simulink model "suspension_3dof"  (R2022b)
settings: Solver=ode45  StartTime=0.0  StopTime=100  MaxStep=0.001  RelTol=1e-3  AbsTol=1e-6
PreLoadFcn:
  | sldemo_suspn_3dof_data
values from neighbouring files (symbols this model uses):
  Cr = 2000    [sldemo_suspn_3dof_data.m]
  g = 9.81    [sldemo_suspn_3dof_data.m]
  Ixx = 1500    [sldemo_suspn_3dof_data.m]
  Iyy = 2100    [sldemo_suspn_3dof_data.m]
  Kf = 28000    [sldemo_suspn_3dof_data.m]
  Kr = 21000    [sldemo_suspn_3dof_data.m]
  L = 1.2    [sldemo_suspn_3dof_data.m]
  Mb = 1200    [sldemo_suspn_3dof_data.m]
  W = 0.9    [sldemo_suspn_3dof_data.m]
libraries: SignalEditorBlockLib x1
CloseFcn:
  | clear Cf Cr Ixx Iyy Kf Kr L Mb W g x0;
Description:
  | Automotive Suspension
  | 
  | This demo describes a simplified car suspension model in three degrees of
  | freedom (DoF): pitch, yaw and vertical displacement. The demo provides a description of the model to
  | show how simulation can be used for investigating ride characteristics. The Signal Editor block was used to
  | capture different road profiles to test the suspension against.
settings Model: FPTRunName=Active  ModifiedByFormat=The MathWorks Inc.  TunableVars=Cf,Mb  TunableVarsStorageClass=Auto,Auto  TunableVarsTypeQualifier=,  Creator=The MathWorks, Inc.  LastModifiedBy=The MathWorks Inc.
settings SolverCC: AutoScaleAbsTol=off  AlgebraicLoopSolver=TrustRegion
settings DataIOCC: InitialState=x0  SaveFormat=Array  SaveOutput=off  DSMLogging=off  SaveTime=off  StateSaveName=x  ReturnWorkspaceOutputsName=simout
settings OptimizationCC: BooleanDataType=off  DefaultParameterBehavior=Inlined  InlineInvariantSignals=on  ExpressionDepthLimit=2147483647  InitFltsAndDblsToZero=on  LifeSpan=inf  BufferReusableBoundary=off
settings DebuggingCC: SaveWithParameterizedLinksMsg=none  SignalResolutionControl=TryResolveAllWithWarning  MultiTaskDSMMsg=warning  SigSpecEnsureSampleTimeMsg=none  IntegerOverflowMsg=none  FcnCallInpInsideContextMsg=warning  UnconnectedInputMsg=warning  UnconnectedOutputMsg=warning  UnconnectedLineMsg=warning  BusObjectLabelMismatch=none  StateNameClashWarn=warning  PregeneratedLibrarySubsystemCodeDiagnostic=none  SFUnexpectedBacktrackingDiag=warning  SFNoUnconditionalDefaultTransitionDiag=warning  SFExecutionAtInitializationDiag=none  SFMachineParentedDataDiag=warning  IntegerSaturationMsg=none  ArithmeticOperatorsInVariantConditions=warning
settings HardwareCC: ProdBitPerPointer=32  ProdBitPerSizeT=32  ProdBitPerPtrDiffT=32  ProdLargestAtomicFloat=None  ProdIntDivRoundTo=Undefined  ProdEndianess=Unspecified  ProdWordSize=32  ProdHWDeviceType=32-bit Generic
settings ModelReferenceCC: EnableRefExpFcnMdlSchedulingChecks=on  PropagateSignalLabelsOutOfModel=off
settings SFSimCC: SimUseLocalCustomCode=off  CustomCodeUndefinedFunction=UseInterfaceOnly
settings RTWCC: RTWUseLocalCustomCode=off  DLArmComputeVersion=19.05
settings CodeAppCC: StateflowObjectComments=on
settings GRTTargetCC: TargetFcnLib=ansi_tfl_tmw.mat  TargetLangStandard=C89/C90 (ANSI)  CombineOutputUpdateFcns=off  GRTInterface=on
settings ConfigComp: CovMetricSettings=dw  CovSaveCumulativeToWorkspaceVar=on  CovSaveSingleToWorkspaceVar=on  CovExternalEMLEnable=off  CovSFcnEnable=off

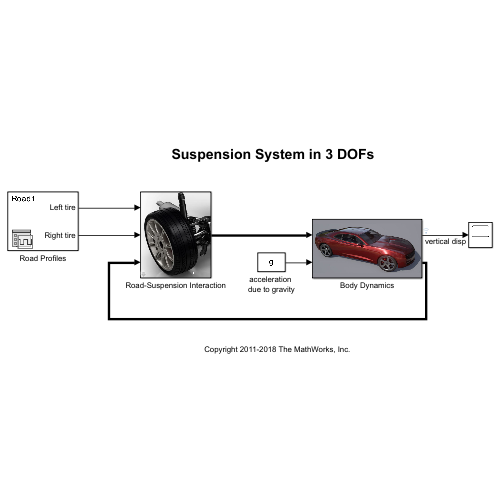
[thumbnail: Simulink's stored preview of the top-level diagram]
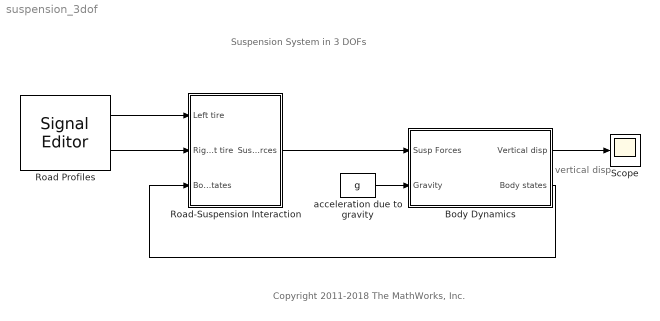
== system suspension_3dof ==
  note: vertical disp
  note: Suspension System in 3 DOFs
  note: Copyright 2011-2018 The MathWorks, Inc.
  Body Dynamics : Subsystem
      mask Display: image('body dynamics.png'); % Use "Edit Image" on toolstrip to change.
  Road Profiles : SignalEditorBlockLib/Signal Editor  FileName=sldemo_suspn_3dof_sigData.mat  ActiveScenario=Road1  ActiveSignal=Left tire  IsBus=off  OutputBusObjectStr=Bus: BusObject  SampleTime=0  OutputAfterFinalValue=Setting to zero  Unit=m  PreserveSignalName=on
  Road-Suspension Interaction : Subsystem  mask{Kf=Kf, Cf=150, Kr=Kr, Cr=Cr}
      mask prompts: Kf "Front susp. stiffness"; Cf "Front susp. damping"; Kr "Rear susp. stiffness"; Cr "Rear susp. damping"
      mask Display: image('road_suspension.png');
  Scope : Scope
  acceleration due to gravity : Constant  Value=g
  wires:
  Road-Suspension Interaction/1(Susp Forces) -> Body Dynamics/1(Susp Forces)
  Road Profiles/1 -> Road-Suspension Interaction/1("Left tire ")
  Road Profiles/2 -> Road-Suspension Interaction/2(Right tire)
  Body Dynamics/2(Body states) -> Road-Suspension Interaction/3(Body States)
  Body Dynamics/1(Vertical disp) -> Scope/1
  acceleration due to gravity/1 -> Body Dynamics/2(Gravity)

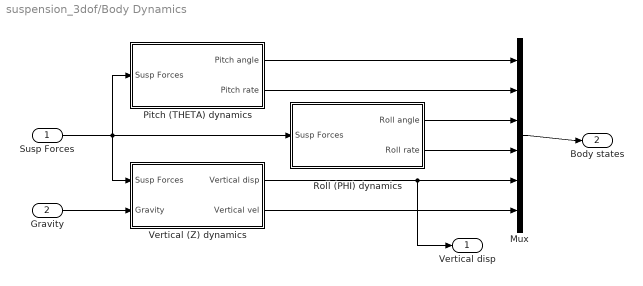
== system suspension_3dof/Body Dynamics ==
  Susp Forces : Inport
  Gravity : Inport  Port=2
  Mux : Mux  Inputs=6
  Pitch (THETA) dynamics : Subsystem
  Roll (PHI) dynamics : Subsystem
  Vertical (Z) dynamics : Subsystem
  Vertical disp : Outport  VectorParamsAs1DForOutWhenUnconnected=off
  Body states : Outport  Port=2  VectorParamsAs1DForOutWhenUnconnected=off
  wires:
  Mux/1 -> Body states/1
  Pitch (THETA) dynamics/1(Pitch angle) -> Mux/1
  Pitch (THETA) dynamics/2(Pitch rate) -> Mux/2
  Roll (PHI) dynamics/1(Roll angle) -> Mux/3
  Roll (PHI) dynamics/2(Roll rate) -> Mux/4
  Vertical (Z) dynamics/1(Vertical disp) -> Mux/5, Vertical disp/1
  Vertical (Z) dynamics/2(Vertical vel) -> Mux/6
  Susp Forces/1 -> Pitch (THETA) dynamics/1(Susp Forces), Roll (PHI) dynamics/1(Susp Forces), Vertical (Z) dynamics/1(Susp Forces)
  Gravity/1 -> Vertical (Z) dynamics/2(Gravity)

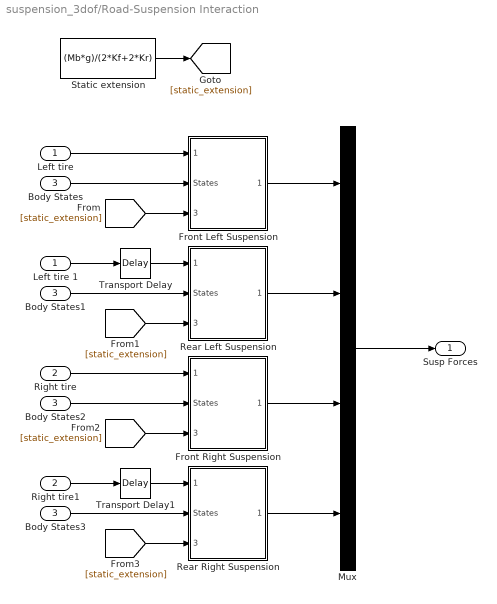
== system suspension_3dof/Road-Suspension Interaction ==
  "Left tire " : Inport
  Right tire : Inport  Port=2
  Body States : Inport  Port=3
  Body States1 : InportShadow  Port=3
  Body States2 : InportShadow  Port=3
  Body States3 : InportShadow  Port=3
  Front Left Suspension : Subsystem  mask(half-car suspension){K=Kf, C=Cf}
      mask prompts: K "Stiffness = spring rate:"; C "Damping rate:"
      mask help:
      | Half-Car Suspension
      | The spring and damping rates for an individual wheel are entered below.  Their combined effect as applied to two wheels at the specified distance from the center of mass is computed.  The distance should be specified as positive if the subsystem is oriented such that increasing z corresponds to increasing theta, negative otherwise.
      mask Help: See "Using Simulink and Stateflow in Automotive Applications" for a mathematical derivation of the subsystem operation.  Contact your MathWorks distributor to obtain a copy.
      mask Display: plot(-1, 0, 13, 12, [1 12], [11 11], [1 5], [2 2], [1 2], [4.5 5], [2 0], [5 6], [0 2], [6 7], [2 0], [7 8], [0 1], [8 8.5], [1 1], [8.5 11], [1 1], [2 4.5], [5 5], [2 5], [4 6], [5 5], [4 4], [5 8], [6 6], [5 8], [4 6], [6.5 6.5], [5 5], [6.5 11], [0 1], [1 2], [2 3], [1 2], [4 5], [1 2])
  Front Right Suspension : Subsystem  mask(half-car suspension){K=Kf, C=Cf}
      mask prompts: K "Stiffness = spring rate:"; C "Damping rate:"
      mask help:
      | Half-Car Suspension
      | The spring and damping rates for an individual wheel are entered below.  Their combined effect as applied to two wheels at the specified distance from the center of mass is computed.  The distance should be specified as positive if the subsystem is oriented such that increasing z corresponds to increasing theta, negative otherwise.
      mask Help: See "Using Simulink and Stateflow in Automotive Applications" for a mathematical derivation of the subsystem operation.  Contact your MathWorks distributor to obtain a copy.
      mask Display: plot(-1, 0, 13, 12, [1 12], [11 11], [1 5], [2 2], [1 2], [4.5 5], [2 0], [5 6], [0 2], [6 7], [2 0], [7 8], [0 1], [8 8.5], [1 1], [8.5 11], [1 1], [2 4.5], [5 5], [2 5], [4 6], [5 5], [4 4], [5 8], [6 6], [5 8], [4 6], [6.5 6.5], [5 5], [6.5 11], [0 1], [1 2], [2 3], [1 2], [4 5], [1 2])
  Left tire 1 : InportShadow
  Mux : Mux
  Rear Left Suspension : Subsystem  mask(half-car suspension){K=Kr, C=Cr}
      mask prompts: K "Stiffness = spring rate:"; C "Damping rate:"
      mask help:
      | Half-Car Suspension
      | The spring and damping rates for an individual wheel are entered below.  Their combined effect as applied to two wheels at the specified distance from the center of mass is computed.  The distance should be specified as positive if the subsystem is oriented such that increasing z corresponds to increasing theta, negative otherwise.
      mask Help: See "Using Simulink and Stateflow in Automotive Applications" for a mathematical derivation of the subsystem operation.  Contact your MathWorks distributor to obtain a copy.
      mask Display: plot(-1, 0, 13, 12, [1 12], [11 11], [1 5], [2 2], [1 2], [4.5 5], [2 0], [5 6], [0 2], [6 7], [2 0], [7 8], [0 1], [8 8.5], [1 1], [8.5 11], [1 1], [2 4.5], [5 5], [2 5], [4 6], [5 5], [4 4], [5 8], [6 6], [5 8], [4 6], [6.5 6.5], [5 5], [6.5 11], [0 1], [1 2], [2 3], [1 2], [4 5], [1 2])
  Rear Right Suspension : Subsystem  mask(half-car suspension){K=Kr, C=Cr}
      mask prompts: K "Stiffness = spring rate:"; C "Damping rate:"
      mask help:
      | Half-Car Suspension
      | The spring and damping rates for an individual wheel are entered below.  Their combined effect as applied to two wheels at the specified distance from the center of mass is computed.  The distance should be specified as positive if the subsystem is oriented such that increasing z corresponds to increasing theta, negative otherwise.
      mask Help: See "Using Simulink and Stateflow in Automotive Applications" for a mathematical derivation of the subsystem operation.  Contact your MathWorks distributor to obtain a copy.
      mask Display: plot(-1, 0, 13, 12, [1 12], [11 11], [1 5], [2 2], [1 2], [4.5 5], [2 0], [5 6], [0 2], [6 7], [2 0], [7 8], [0 1], [8 8.5], [1 1], [8.5 11], [1 1], [2 4.5], [5 5], [2 5], [4 6], [5 5], [4 4], [5 8], [6 6], [5 8], [4 6], [6.5 6.5], [5 5], [6.5 11], [0 1], [1 2], [2 3], [1 2], [4 5], [1 2])
  Right tire1 : InportShadow  Port=2
  Static extension : Constant  Value=(Mb*g)/(2*Kf+2*Kr)
  Transport Delay : TransportDelay  DelayTime=0.1
  Transport Delay1 : TransportDelay  DelayTime=0.1
  Susp Forces : Outport  VectorParamsAs1DForOutWhenUnconnected=off
  wires:
  Front Left Suspension/1(Vertical Force) -> Mux/1
  Front Right Suspension/1(Vertical Force) -> Mux/3
  Rear Left Suspension/1(Vertical Force) -> Mux/2
  Rear Right Suspension/1(Vertical Force) -> Mux/4
  "Left tire "/1 -> Front Left Suspension/1(Road Input)
  Mux/1 -> Susp Forces/1
  Left tire 1/1 -> Transport Delay/1
  Right tire1/1 -> Transport Delay1/1
  Body States/1 -> Front Left Suspension/2(States)
  Body States2/1 -> Front Right Suspension/2(States)
  Body States1/1 -> Rear Left Suspension/2(States)
  Transport Delay/1 -> Rear Left Suspension/1(Road Input)
  Right tire/1 -> Front Right Suspension/1(Road Input)
  Transport Delay1/1 -> Rear Right Suspension/1(Road Input)
  Body States3/1 -> Rear Right Suspension/2(States)
  Static extension/1 -> [static_extension]
  [static_extension] -> Front Left Suspension/3(Static ext.)
  [static_extension] -> Front Right Suspension/3(Static ext.)
  [static_extension] -> Rear Right Suspension/3(Static Ext.)
  [static_extension] -> Rear Left Suspension/3(Static Ext.)

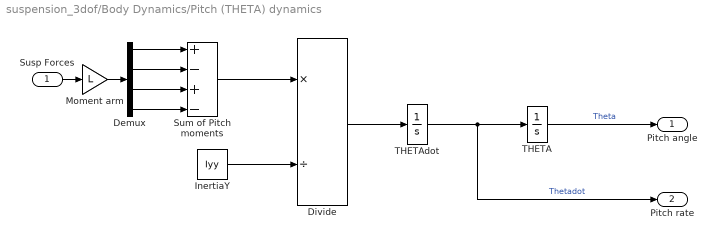
== system suspension_3dof/Body Dynamics/Pitch (THETA) dynamics ==
  Susp Forces : Inport
  Demux : Demux
  Divide : Product  Inputs=*/
  InertiaY : Constant  Value=Iyy
  Moment arm : Gain  Gain=L
  Sum of Pitch moments : Sum  Inputs=+-+-
  THETA : Integrator  InitialCondition=-8.7e-20
  THETAdot : Integrator  InitialCondition=8.04e-28
  Pitch angle : Outport  VectorParamsAs1DForOutWhenUnconnected=off
  Pitch rate : Outport  Port=2  VectorParamsAs1DForOutWhenUnconnected=off
  wires:
  Divide/1 -> THETAdot/1
  THETAdot/1 -> THETA/1, Pitch rate/1  "Thetadot"
  Sum of Pitch moments/1 -> Divide/1
  THETA/1 -> Pitch angle/1  "Theta"
  Susp Forces/1 -> Moment arm/1
  Moment arm/1 -> Demux/1
  Demux/1 -> Sum of Pitch moments/1
  Demux/2 -> Sum of Pitch moments/2
  Demux/3 -> Sum of Pitch moments/3
  Demux/4 -> Sum of Pitch moments/4
  InertiaY/1 -> Divide/2

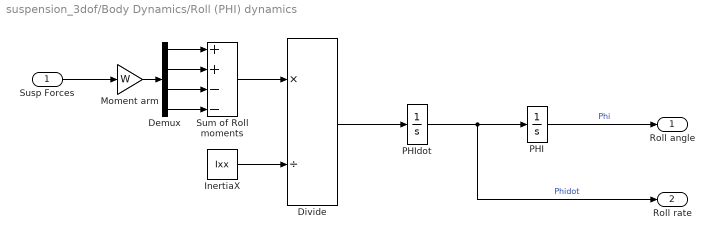
== system suspension_3dof/Body Dynamics/Roll (PHI) dynamics ==
  Susp Forces : Inport
  Demux : Demux
  Divide : Product  Inputs=*/
  InertiaX : Constant  Value=Ixx
  Moment arm : Gain  Gain=W
  PHI : Integrator  InitialCondition=-8.7e-20
  PHIdot : Integrator  InitialCondition=8.04e-28
  Sum of Roll moments : Sum  Inputs=++--
  Roll angle : Outport  VectorParamsAs1DForOutWhenUnconnected=off
  Roll rate : Outport  Port=2  VectorParamsAs1DForOutWhenUnconnected=off
  wires:
  PHI/1 -> Roll angle/1  "Phi"
  PHIdot/1 -> Roll rate/1, PHI/1  "Phidot"
  Divide/1 -> PHIdot/1
  Moment arm/1 -> Demux/1
  Susp Forces/1 -> Moment arm/1
  Demux/1 -> Sum of Roll moments/1
  Demux/2 -> Sum of Roll moments/2
  Demux/3 -> Sum of Roll moments/3
  Demux/4 -> Sum of Roll moments/4
  Sum of Roll moments/1 -> Divide/1
  InertiaX/1 -> Divide/2

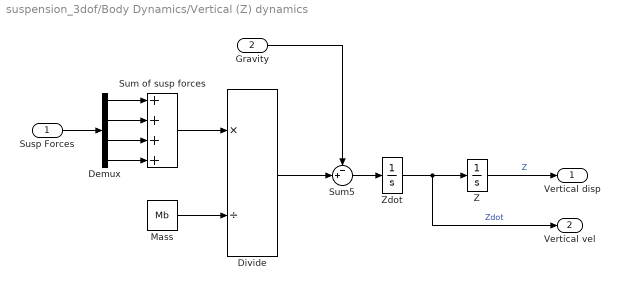
== system suspension_3dof/Body Dynamics/Vertical (Z) dynamics ==
  Susp Forces : Inport
  Gravity : Inport  Port=2
  Demux : Demux
  Divide : Product  Inputs=*/
  Mass : Constant  Value=Mb
  Sum of susp forces : Sum  Inputs=++++
  Sum5 : Sum  Inputs=-+|  InputSameDT=on  SaturateOnIntegerOverflow=on  OutDataTypeStr=Inherit: Same as first input
  Z : Integrator
  Zdot : Integrator
  Vertical disp : Outport  VectorParamsAs1DForOutWhenUnconnected=off
  Vertical vel : Outport  Port=2  VectorParamsAs1DForOutWhenUnconnected=off
  wires:
  Sum5/1 -> Zdot/1
  Zdot/1 -> Vertical vel/1, Z/1  "Zdot"
  Z/1 -> Vertical disp/1  "Z"
  Susp Forces/1 -> Demux/1
  Demux/1 -> Sum of susp forces/1
  Demux/2 -> Sum of susp forces/2
  Demux/3 -> Sum of susp forces/3
  Demux/4 -> Sum of susp forces/4
  Sum of susp forces/1 -> Divide/1
  Divide/1 -> Sum5/2
  Gravity/1 -> Sum5/1
  Mass/1 -> Divide/2

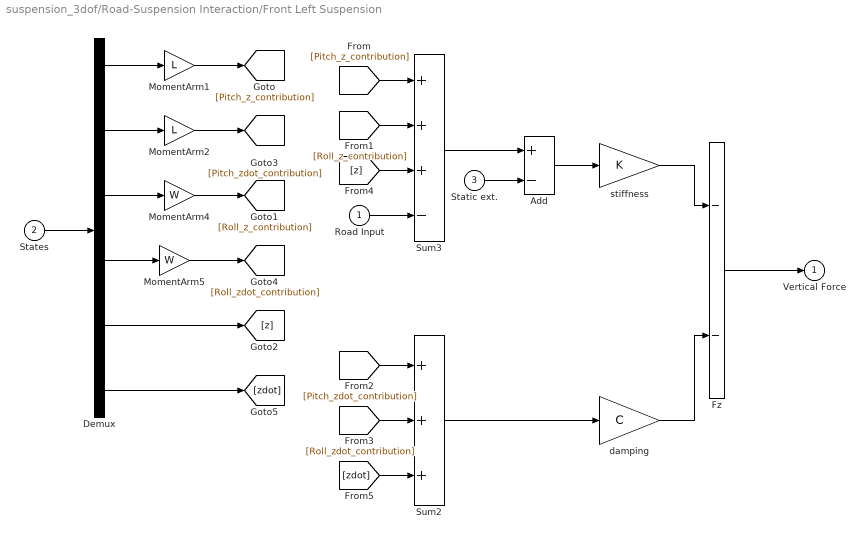
== system suspension_3dof/Road-Suspension Interaction/Front Left Suspension ==
  Road Input : Inport
  States : Inport  Port=2
  Static ext. : Inport  Port=3
  Add : Sum  Inputs=+-
  Demux : Demux  Outputs=6
      settings: DisplayOption=none
  Fz : Sum  Inputs=--  InputSameDT=on  SaturateOnIntegerOverflow=on  OutDataTypeStr=Inherit: Same as first input
  MomentArm1 : Gain  Gain=L  SaturateOnIntegerOverflow=on  OutDataTypeStr=Inherit: Same as input  ParamDataTypeStr=Inherit: Same as input
  MomentArm2 : Gain  Gain=L  SaturateOnIntegerOverflow=on  OutDataTypeStr=Inherit: Same as input  ParamDataTypeStr=Inherit: Same as input
  MomentArm4 : Gain  Gain=W  SaturateOnIntegerOverflow=on  OutDataTypeStr=Inherit: Same as input  ParamDataTypeStr=Inherit: Same as input
  MomentArm5 : Gain  Gain=W  SaturateOnIntegerOverflow=on  OutDataTypeStr=Inherit: Same as input  ParamDataTypeStr=Inherit: Same as input
  Sum2 : Sum  Inputs=+++  InputSameDT=on  SaturateOnIntegerOverflow=on  OutDataTypeStr=Inherit: Same as first input
  Sum3 : Sum  Inputs=+++-  InputSameDT=on  SaturateOnIntegerOverflow=on  OutDataTypeStr=Inherit: Same as first input
  damping : Gain  Gain=C  SaturateOnIntegerOverflow=on  OutDataTypeStr=Inherit: Same as input  ParamDataTypeStr=Inherit: Same as input
  stiffness : Gain  Gain=K  SaturateOnIntegerOverflow=on  OutDataTypeStr=Inherit: Same as input  ParamDataTypeStr=Inherit: Same as input
  Vertical Force : Outport  VectorParamsAs1DForOutWhenUnconnected=off
  wires:
  Sum2/1 -> damping/1
  States/1 -> Demux/1
  damping/1 -> Fz/2
  stiffness/1 -> Fz/1
  Demux/1 -> MomentArm1/1
  Demux/2 -> MomentArm2/1
  Fz/1 -> Vertical Force/1
  Demux/3 -> MomentArm4/1
  Demux/4 -> MomentArm5/1
  Sum3/1 -> Add/1
  Add/1 -> stiffness/1
  MomentArm1/1 -> [Pitch_z_contribution]
  MomentArm4/1 -> [Roll_z_contribution]
  Demux/5 -> [z]
  MomentArm2/1 -> [Pitch_zdot_contribution]
  MomentArm5/1 -> [Roll_zdot_contribution]
  Demux/6 -> [zdot]
  [Pitch_zdot_contribution] -> Sum2/1
  [Roll_zdot_contribution] -> Sum2/2
  [Pitch_z_contribution] -> Sum3/1
  [Roll_z_contribution] -> Sum3/2
  [z] -> Sum3/3
  [zdot] -> Sum2/3
  Road Input/1 -> Sum3/4
  Static ext./1 -> Add/2

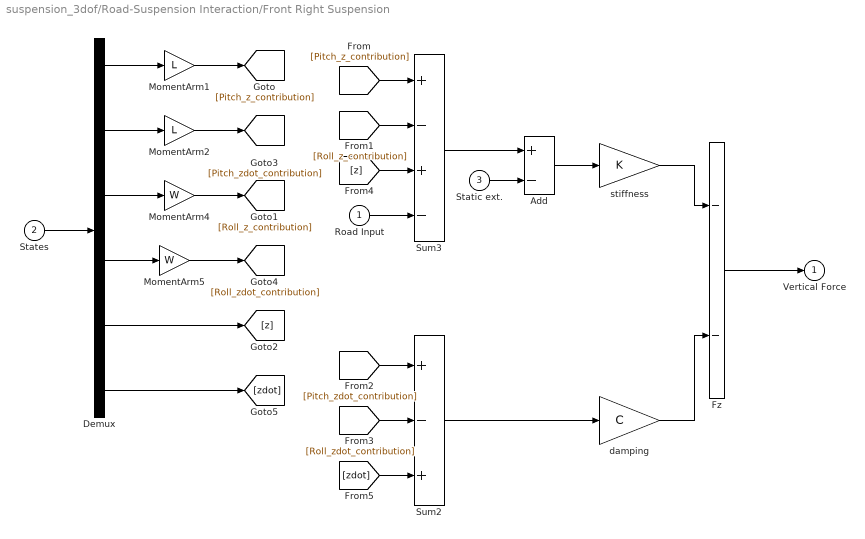
== system suspension_3dof/Road-Suspension Interaction/Front Right Suspension ==
  Road Input : Inport
  States : Inport  Port=2
  Static ext. : Inport  Port=3
  Add : Sum  Inputs=+-
  Demux : Demux  Outputs=6
      settings: DisplayOption=none
  Fz : Sum  Inputs=--  InputSameDT=on  SaturateOnIntegerOverflow=on  OutDataTypeStr=Inherit: Same as first input
  MomentArm1 : Gain  Gain=L  SaturateOnIntegerOverflow=on  OutDataTypeStr=Inherit: Same as input  ParamDataTypeStr=Inherit: Same as input
  MomentArm2 : Gain  Gain=L  SaturateOnIntegerOverflow=on  OutDataTypeStr=Inherit: Same as input  ParamDataTypeStr=Inherit: Same as input
  MomentArm4 : Gain  Gain=W  SaturateOnIntegerOverflow=on  OutDataTypeStr=Inherit: Same as input  ParamDataTypeStr=Inherit: Same as input
  MomentArm5 : Gain  Gain=W  SaturateOnIntegerOverflow=on  OutDataTypeStr=Inherit: Same as input  ParamDataTypeStr=Inherit: Same as input
  Sum2 : Sum  Inputs=+-+  InputSameDT=on  SaturateOnIntegerOverflow=on  OutDataTypeStr=Inherit: Same as first input
  Sum3 : Sum  Inputs=+-+-  InputSameDT=on  SaturateOnIntegerOverflow=on  OutDataTypeStr=Inherit: Same as first input
  damping : Gain  Gain=C  SaturateOnIntegerOverflow=on  OutDataTypeStr=Inherit: Same as input  ParamDataTypeStr=Inherit: Same as input
  stiffness : Gain  Gain=K  SaturateOnIntegerOverflow=on  OutDataTypeStr=Inherit: Same as input  ParamDataTypeStr=Inherit: Same as input
  Vertical Force : Outport  VectorParamsAs1DForOutWhenUnconnected=off
  wires:
  Sum2/1 -> damping/1
  States/1 -> Demux/1
  damping/1 -> Fz/2
  stiffness/1 -> Fz/1
  Demux/1 -> MomentArm1/1
  Demux/2 -> MomentArm2/1
  Fz/1 -> Vertical Force/1
  Demux/3 -> MomentArm4/1
  Demux/4 -> MomentArm5/1
  Sum3/1 -> Add/1
  Add/1 -> stiffness/1
  MomentArm1/1 -> [Pitch_z_contribution]
  MomentArm4/1 -> [Roll_z_contribution]
  Demux/5 -> [z]
  MomentArm2/1 -> [Pitch_zdot_contribution]
  MomentArm5/1 -> [Roll_zdot_contribution]
  Demux/6 -> [zdot]
  [Pitch_zdot_contribution] -> Sum2/1
  [Roll_zdot_contribution] -> Sum2/2
  [Pitch_z_contribution] -> Sum3/1
  [Roll_z_contribution] -> Sum3/2
  [z] -> Sum3/3
  [zdot] -> Sum2/3
  Road Input/1 -> Sum3/4
  Static ext./1 -> Add/2

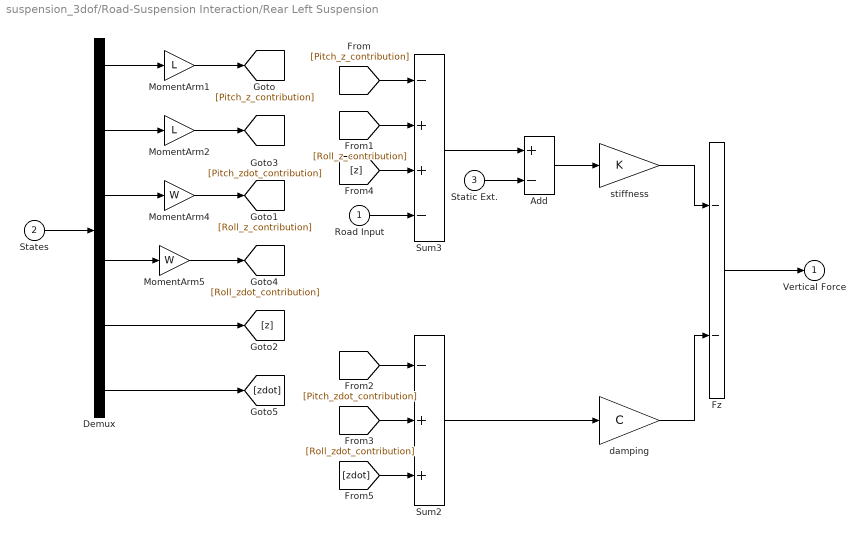
== system suspension_3dof/Road-Suspension Interaction/Rear Left Suspension ==
  Road Input : Inport
  States : Inport  Port=2
  Static Ext. : Inport  Port=3
  Add : Sum  Inputs=+-
  Demux : Demux  Outputs=6
      settings: DisplayOption=none
  Fz : Sum  Inputs=--  InputSameDT=on  SaturateOnIntegerOverflow=on  OutDataTypeStr=Inherit: Same as first input
  MomentArm1 : Gain  Gain=L  SaturateOnIntegerOverflow=on  OutDataTypeStr=Inherit: Same as input  ParamDataTypeStr=Inherit: Same as input
  MomentArm2 : Gain  Gain=L  SaturateOnIntegerOverflow=on  OutDataTypeStr=Inherit: Same as input  ParamDataTypeStr=Inherit: Same as input
  MomentArm4 : Gain  Gain=W  SaturateOnIntegerOverflow=on  OutDataTypeStr=Inherit: Same as input  ParamDataTypeStr=Inherit: Same as input
  MomentArm5 : Gain  Gain=W  SaturateOnIntegerOverflow=on  OutDataTypeStr=Inherit: Same as input  ParamDataTypeStr=Inherit: Same as input
  Sum2 : Sum  Inputs=-++  InputSameDT=on  SaturateOnIntegerOverflow=on  OutDataTypeStr=Inherit: Same as first input
  Sum3 : Sum  Inputs=-++-  InputSameDT=on  SaturateOnIntegerOverflow=on  OutDataTypeStr=Inherit: Same as first input
  damping : Gain  Gain=C  SaturateOnIntegerOverflow=on  OutDataTypeStr=Inherit: Same as input  ParamDataTypeStr=Inherit: Same as input
  stiffness : Gain  Gain=K  SaturateOnIntegerOverflow=on  OutDataTypeStr=Inherit: Same as input  ParamDataTypeStr=Inherit: Same as input
  Vertical Force : Outport  VectorParamsAs1DForOutWhenUnconnected=off
  wires:
  Road Input/1 -> Sum3/4
  [zdot] -> Sum2/3
  [z] -> Sum3/3
  [Roll_z_contribution] -> Sum3/2
  [Pitch_z_contribution] -> Sum3/1
  [Roll_zdot_contribution] -> Sum2/2
  [Pitch_zdot_contribution] -> Sum2/1
  Demux/6 -> [zdot]
  MomentArm5/1 -> [Roll_zdot_contribution]
  MomentArm2/1 -> [Pitch_zdot_contribution]
  Demux/5 -> [z]
  MomentArm4/1 -> [Roll_z_contribution]
  MomentArm1/1 -> [Pitch_z_contribution]
  Add/1 -> stiffness/1
  Sum3/1 -> Add/1
  Demux/4 -> MomentArm5/1
  Demux/3 -> MomentArm4/1
  Fz/1 -> Vertical Force/1
  Demux/2 -> MomentArm2/1
  Demux/1 -> MomentArm1/1
  stiffness/1 -> Fz/1
  damping/1 -> Fz/2
  States/1 -> Demux/1
  Sum2/1 -> damping/1
  Static Ext./1 -> Add/2

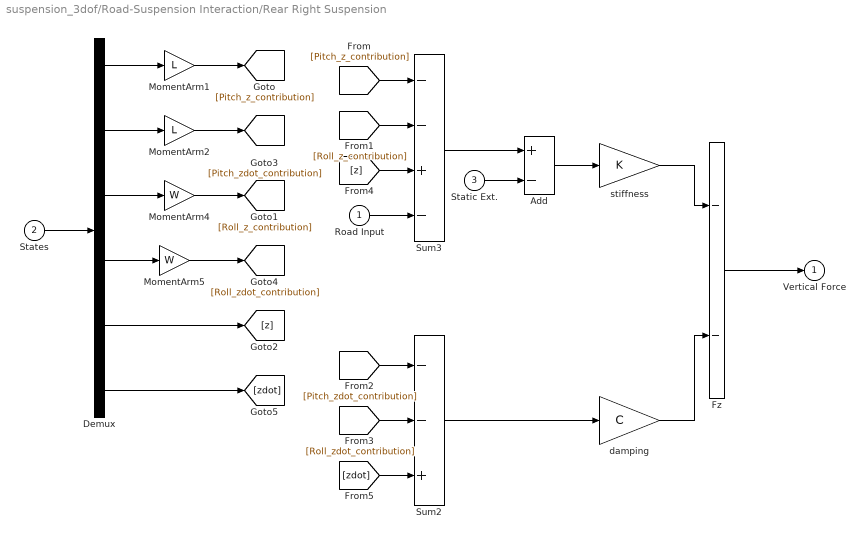
== system suspension_3dof/Road-Suspension Interaction/Rear Right Suspension ==
  Road Input : Inport
  States : Inport  Port=2
  Static Ext. : Inport  Port=3
  Add : Sum  Inputs=+-
  Demux : Demux  Outputs=6
      settings: DisplayOption=none
  Fz : Sum  Inputs=--  InputSameDT=on  SaturateOnIntegerOverflow=on  OutDataTypeStr=Inherit: Same as first input
  MomentArm1 : Gain  Gain=L  SaturateOnIntegerOverflow=on  OutDataTypeStr=Inherit: Same as input  ParamDataTypeStr=Inherit: Same as input
  MomentArm2 : Gain  Gain=L  SaturateOnIntegerOverflow=on  OutDataTypeStr=Inherit: Same as input  ParamDataTypeStr=Inherit: Same as input
  MomentArm4 : Gain  Gain=W  SaturateOnIntegerOverflow=on  OutDataTypeStr=Inherit: Same as input  ParamDataTypeStr=Inherit: Same as input
  MomentArm5 : Gain  Gain=W  SaturateOnIntegerOverflow=on  OutDataTypeStr=Inherit: Same as input  ParamDataTypeStr=Inherit: Same as input
  Sum2 : Sum  Inputs=--+  InputSameDT=on  SaturateOnIntegerOverflow=on  OutDataTypeStr=Inherit: Same as first input
  Sum3 : Sum  Inputs=--+-  InputSameDT=on  SaturateOnIntegerOverflow=on  OutDataTypeStr=Inherit: Same as first input
  damping : Gain  Gain=C  SaturateOnIntegerOverflow=on  OutDataTypeStr=Inherit: Same as input  ParamDataTypeStr=Inherit: Same as input
  stiffness : Gain  Gain=K  SaturateOnIntegerOverflow=on  OutDataTypeStr=Inherit: Same as input  ParamDataTypeStr=Inherit: Same as input
  Vertical Force : Outport  VectorParamsAs1DForOutWhenUnconnected=off
  wires:
  Road Input/1 -> Sum3/4
  [zdot] -> Sum2/3
  [z] -> Sum3/3
  [Roll_z_contribution] -> Sum3/2
  [Pitch_z_contribution] -> Sum3/1
  [Roll_zdot_contribution] -> Sum2/2
  [Pitch_zdot_contribution] -> Sum2/1
  Demux/6 -> [zdot]
  MomentArm5/1 -> [Roll_zdot_contribution]
  MomentArm2/1 -> [Pitch_zdot_contribution]
  Demux/5 -> [z]
  MomentArm4/1 -> [Roll_z_contribution]
  MomentArm1/1 -> [Pitch_z_contribution]
  Add/1 -> stiffness/1
  Sum3/1 -> Add/1
  Demux/4 -> MomentArm5/1
  Demux/3 -> MomentArm4/1
  Fz/1 -> Vertical Force/1
  Demux/2 -> MomentArm2/1
  Demux/1 -> MomentArm1/1
  stiffness/1 -> Fz/1
  damping/1 -> Fz/2
  States/1 -> Demux/1
  Sum2/1 -> damping/1
  Static Ext./1 -> Add/2
